simulink model "mcb_pmsm_hall_offset_f28069m"  (R2024b)
settings: Solver=FixedStepDiscrete  StartTime=0.0  StopTime=2  RelTol=1e-3  EnableMultiTasking=on
InitFcn:
  | mcb_pmsm_offset_data;
  | target = mcb_SetProcessorDetails('F28069M',PWM_frequency);
undefined symbols (not defined in the file): Down, GPTRIP1SEL, GPTRIP2SEL, motor, PWM_frequency, Ts, TZ1, TZ2, Up
libraries: simulink x8, idelinklib_common x6, svdschedulerlib x5, c280xlib x5, mcbcontrolslib x5, mcbpositiondecoderlib x4, c2802xlib x4, c2806xlib x2
(part 2 of 2)

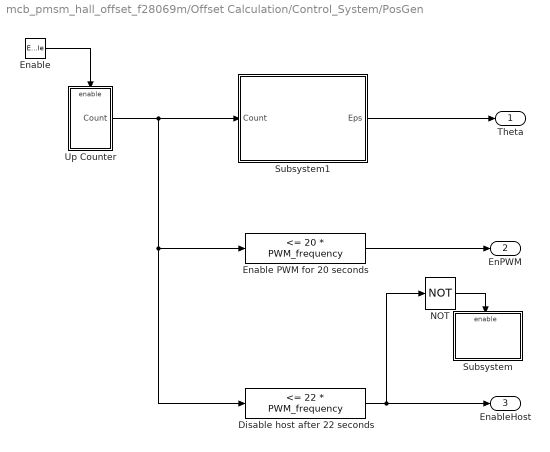
== system mcb_pmsm_hall_offset_f28069m/Offset Calculation/Control_System/PosGen ==
  Enable : EnablePort  StatesWhenEnabling=reset  ShowOutputPort=on
  Disable host after 22 seconds : simulink/Logic and Bit Operations/Compare To Constant  relop=<=  const=22 * PWM_frequency  OutDataTypeStr=boolean
  Enable PWM for 20 seconds : simulink/Logic and Bit Operations/Compare To Constant  relop=<=  const=20 * PWM_frequency  OutDataTypeStr=boolean
  NOT : Logic  Operator=NOT  IconShape=distinctive  AllPortsSameDT=off  OutDataTypeStr=boolean
  Subsystem : Subsystem
  Subsystem1 : Subsystem
  Up Counter : Subsystem
  Theta : Outport
  EnPWM : Outport  Port=2  OutputWhenDisabled=reset  InitialOutput=0  VectorParamsAs1DForOutWhenUnconnected=off
  EnableHost : Outport  Port=3  OutputWhenDisabled=reset  InitialOutput=0  VectorParamsAs1DForOutWhenUnconnected=off
  wires:
  Subsystem1/1(Eps) -> Theta/1
  Up Counter/1(Count) -> Disable host after 22 seconds/1, Enable PWM for 20 seconds/1, Subsystem1/1(Count)
  Enable/1 -> Up Counter/Enable
  NOT/1 -> Subsystem/Enable
  Enable PWM for 20 seconds/1 -> EnPWM/1
  Disable host after 22 seconds/1 -> NOT/1, EnableHost/1

== system mcb_pmsm_hall_offset_f28069m/Offset Calculation/Control_System/Subsystem1 ==
  Input : Inport
  Enable : EnablePort
  Offset : Outport
  wires:
  Input/1 -> Offset/1

== system mcb_pmsm_hall_offset_f28069m/Offset Calculation/Data Serial Output/Data ==
  Data : Inport
  Data_width : Inport  Port=2
  Action Port : ActionPort  ActionPortLabel=else
  Mux : Mux  Inputs=2
  Start : Constant  Value=hex2dec('0000')  OutDataTypeStr=uint16
  Data_out : Outport  VectorParamsAs1DForOutWhenUnconnected=off
  Iteration : Outport  Port=2  VectorParamsAs1DForOutWhenUnconnected=off
  wires:
  Start/1 -> Mux/2
  Mux/1 -> Data_out/1
  Data/1 -> Mux/1
  Data_width/1 -> Iteration/1

== system mcb_pmsm_hall_offset_f28069m/Offset Calculation/Data Serial Output/Data_Conditioning ==
  In1 : Inport
  Data Type Conversion1 : DataTypeConversion  OutDataTypeStr=fixdt(1,32,12)  RndMeth=Simplest  SaturateOnIntegerOverflow=off
  Data Type Conversion3 : DataTypeConversion  OutDataTypeStr=uint16  ConvertRealWorld=Stored Integer (SI)  SaturateOnIntegerOverflow=off  RndMeth=Floor
  Out1 : Outport
  wires:
  Data Type Conversion1/1 -> Data Type Conversion3/1
  In1/1 -> Data Type Conversion1/1
  Data Type Conversion3/1 -> Out1/1

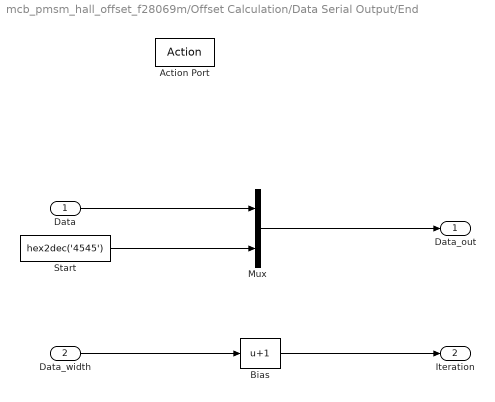
== system mcb_pmsm_hall_offset_f28069m/Offset Calculation/Data Serial Output/End ==
  Data : Inport
  Data_width : Inport  Port=2
  Action Port : ActionPort  ActionPortLabel=elseif(u1 == 599)
  Bias : Bias  Bias=1  SaturateOnIntegerOverflow=off
  Mux : Mux  Inputs=2
  Start : Constant  Value=hex2dec('4545')  OutDataTypeStr=uint16
  Data_out : Outport  VectorParamsAs1DForOutWhenUnconnected=off
  Iteration : Outport  Port=2  VectorParamsAs1DForOutWhenUnconnected=off
  wires:
  Mux/1 -> Data_out/1
  Data_width/1 -> Bias/1
  Start/1 -> Mux/2
  Bias/1 -> Iteration/1
  Data/1 -> Mux/1

== system mcb_pmsm_hall_offset_f28069m/Offset Calculation/Data Serial Output/Start ==
  Data : Inport
  Data_width : Inport  Port=2
  Action Port : ActionPort  ActionPortLabel=if(u1 == 0)
  Bias : Bias  Bias=1  SaturateOnIntegerOverflow=off
  End : Constant  Value=hex2dec('5353')  OutDataTypeStr=uint16
  Mux : Mux  Inputs=2
  Data_out : Outport  VectorParamsAs1DForOutWhenUnconnected=off
  Iteration : Outport  Port=2  VectorParamsAs1DForOutWhenUnconnected=off
  wires:
  End/1 -> Mux/1
  Mux/1 -> Data_out/1
  Data_width/1 -> Bias/1
  Bias/1 -> Iteration/1
  Data/1 -> Mux/2

== system mcb_pmsm_hall_offset_f28069m/Offset Calculation/Data Serial Output/While Iterator Subsystem ==
  Data : Inport
  Iteration : Inport  Port=2
  Add : Sum  Inputs=+-  OutDataTypeStr=Inherit: Same as first input
  Index Vector : MultiPortSwitch  Inputs=1  SaturateOnIntegerOverflow=off  InputSameDT=off
  SCI Transmit : c280xlib/SCI Transmit  sciModule=A  dataHead=''  dataTail=''  frameSize=1  blockingMode=on  outputStatus=off
  While Iterator : WhileIterator  MaxIters=-1  WhileBlockType=do-while  ShowIterationPort=on  OutputDataType=int16
  wires:
  Iteration/1 -> Add/1
  Add/1 -> While Iterator/1
  Index Vector/1 -> SCI Transmit/1
  Data/1 -> Index Vector/2
  While Iterator/1 -> Index Vector/1, Add/2

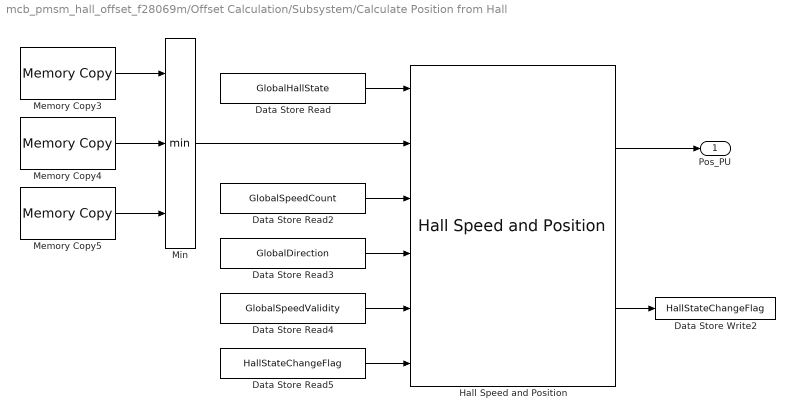
== system mcb_pmsm_hall_offset_f28069m/Offset Calculation/Subsystem/Calculate Position from Hall ==
  Data Store Read : DataStoreRead  DataStoreName=GlobalHallState  IndexOptions=Index vector (dialog)  Indices=1  OutputSizes=1
  Data Store Read2 : DataStoreRead  DataStoreName=GlobalSpeedCount  IndexOptions=Index vector (dialog)  Indices=1  OutputSizes=1
  Data Store Read3 : DataStoreRead  DataStoreName=GlobalDirection  IndexOptions=Index vector (dialog)  Indices=1  OutputSizes=1
  Data Store Read4 : DataStoreRead  DataStoreName=GlobalSpeedValidity  IndexOptions=Index vector (dialog)  Indices=1  OutputSizes=1
  Data Store Read5 : DataStoreRead  Priority=1  DataStoreName=HallStateChangeFlag  IndexOptions=Index vector (dialog)  Indices=1  OutputSizes=1
  Data Store Write2 : DataStoreWrite  Priority=2  DataStoreName=HallStateChangeFlag  IndexOptions=Index vector (dialog)  Indices=1  OutputSizes=1
  Hall Speed and Position : mcbpositiondecoderlib/Hall Speed and Position  blkExecutionType=Position  CounterSize=32 bits  ClkFreq=target.CPU_frequency  BlkSampleTime=Ts  PolePairs=motor.polePairs  MinSpeed=20  HallInterruptConfig=Every 180 Degrees  SpeedUnit=Per unit  PerUnitSpeed=6000  SpeedDataType=dataType  hallSequence=ABC  Sequence=[5,4,6,2,3,1]  EnableSecondOrder=1st Order  PositionUnit=Per unit  PositionDataType=dataType
  Memory Copy3 : idelinklib_common/Memory Copy  copyFrom=Specified source code symbol  copyFromAddressSource=Specify via dialog  copyFromAddress=hex2dec('00001000')  copyFromSrcCode=&ECap1Regs.TSCTR  dataTypeFrom=uint32  dataDimensionFrom=1  useOffsetFrom=off  offsetFromSrc=Specify via dialog  offsetFrom=0  strideFrom=1  copyTo=Output port  copyToAddressSource=Specify via dialog  copyToAddress=hex2dec('00002000')  copyToSrcCode=myVariableDst  dataTypeTo=uint32  useOffsetTo=off  offsetToSrc=Specify via dialog  offsetTo=0  strideTo=1  sampleTime=-1  useInitValue=off  initValueSrc=Specify constant value  initValue=1  initValueSrcCode=myInitValueVariable  useAsMask=off  maskOperator=bitwise AND  useTermValue=off  termValue=1  isRealtimeEnabled=off  emitCCBeforeWrite=off  CCBeforeWrite=/* Custom Code Before Write*/  emitCCAfterWrite=off  CCAfterWrite=/* Custom Code After Write*/
  Memory Copy4 : idelinklib_common/Memory Copy  copyFrom=Specified source code symbol  copyFromAddressSource=Specify via dialog  copyFromAddress=hex2dec('00001000')  copyFromSrcCode=&ECap2Regs.TSCTR  dataTypeFrom=uint32  dataDimensionFrom=1  useOffsetFrom=off  offsetFromSrc=Specify via dialog  offsetFrom=0  strideFrom=1  copyTo=Output port  copyToAddressSource=Specify via dialog  copyToAddress=hex2dec('00002000')  copyToSrcCode=myVariableDst  dataTypeTo=uint32  useOffsetTo=off  offsetToSrc=Specify via dialog  offsetTo=0  strideTo=1  sampleTime=-1  useInitValue=off  initValueSrc=Specify constant value  initValue=1  initValueSrcCode=myInitValueVariable  useAsMask=off  maskOperator=bitwise AND  useTermValue=off  termValue=1  isRealtimeEnabled=off  emitCCBeforeWrite=off  CCBeforeWrite=/* Custom Code Before Write*/  emitCCAfterWrite=off  CCAfterWrite=/* Custom Code After Write*/
  Memory Copy5 : idelinklib_common/Memory Copy  copyFrom=Specified source code symbol  copyFromAddressSource=Specify via dialog  copyFromAddress=hex2dec('00001000')  copyFromSrcCode=&ECap3Regs.TSCTR  dataTypeFrom=uint32  dataDimensionFrom=1  useOffsetFrom=off  offsetFromSrc=Specify via dialog  offsetFrom=0  strideFrom=1  copyTo=Output port  copyToAddressSource=Specify via dialog  copyToAddress=hex2dec('00002000')  copyToSrcCode=myVariableDst  dataTypeTo=uint32  useOffsetTo=off  offsetToSrc=Specify via dialog  offsetTo=0  strideTo=1  sampleTime=-1  useInitValue=off  initValueSrc=Specify constant value  initValue=1  initValueSrcCode=myInitValueVariable  useAsMask=off  maskOperator=bitwise AND  useTermValue=off  termValue=1  isRealtimeEnabled=off  emitCCBeforeWrite=off  CCBeforeWrite=/* Custom Code Before Write*/  emitCCAfterWrite=off  CCAfterWrite=/* Custom Code After Write*/
  Min : MinMax  Inputs=3
  Pos_PU : Outport  InitialOutput=0  VectorParamsAs1DForOutWhenUnconnected=off
  wires:
  Hall Speed and Position/2 -> Data Store Write2/1
  Data Store Read/1 -> Hall Speed and Position/1
  Data Store Read5/1 -> Hall Speed and Position/6
  Data Store Read4/1 -> Hall Speed and Position/5
  Memory Copy4/1 -> Min/2
  Min/1 -> Hall Speed and Position/2
  Memory Copy3/1 -> Min/1
  Data Store Read2/1 -> Hall Speed and Position/3
  Data Store Read3/1 -> Hall Speed and Position/4
  Memory Copy5/1 -> Min/3
  Hall Speed and Position/1 -> Pos_PU/1

== system mcb_pmsm_hall_offset_f28069m/Offset Calculation/Control_System/Find Offset/Subsystem ==
  Theta_hall : Inport
  Enable : EnablePort
  IIR Filter : mcbcontrolslib/IIR Filter  VariantControl=Low Pass Filter  VariantSelect=Low-pass  FilterConstantInputType=Specify via dialog  Filter_constant=0.5  advancedSettings=off  Ts=50e-6  cutOff_freq=3183.0989
  Offset : Outport
  wires:
  IIR Filter/1 -> Offset/1
  Theta_hall/1 -> IIR Filter/1

== system mcb_pmsm_hall_offset_f28069m/Offset Calculation/Control_System/PosGen/Subsystem ==
  Enable : EnablePort
  Constant : Constant  Value=0  OutDataTypeStr=Inherit: Inherit via back propagation
  Data Store Write : DataStoreWrite  DataStoreName=Enable  IndexOptions=Index vector (dialog)  Indices=1  OutputSizes=1
  wires:
  Constant/1 -> Data Store Write/1

== system mcb_pmsm_hall_offset_f28069m/Offset Calculation/Control_System/PosGen/Subsystem1 ==
  Count : Inport
  Count for 2 sec : Constant  Value=2.5 * PWM_frequency  OutDataTypeStr=uint32  SampleTime=-1
  If : If  NumInputs=2  IfExpression=u1 < u2
  If Action Subsystem : Subsystem  TreatAsAtomicUnit=on
  If Action Subsystem2 : Subsystem  TreatAsAtomicUnit=on
  Merge : Merge
  Position Generator : mcbcontrolslib/Position Generator  AngleOutput=Per-unit  ExternalReset=none  Offset=0
  Eps : Outport
  wires:
  If Action Subsystem/1(Out1) -> Merge/1
  If/1 -> If Action Subsystem/Action
  If Action Subsystem2/1(Out1) -> Merge/2
  Position Generator/1 -> Eps/1  "Eps"
  Count/1 -> If/1
  Merge/1 -> Position Generator/1
  If/2 -> If Action Subsystem2/Action
  Count for 2 sec/1 -> If/2

== system mcb_pmsm_hall_offset_f28069m/Offset Calculation/Control_System/PosGen/Up Counter ==
  Enable : EnablePort  StatesWhenEnabling=reset
  Add1 : Sum  SaturateOnIntegerOverflow=on
  Constant : Constant  OutDataTypeStr=uint32
  Delay : Delay  DelayLength=1
  Count : Outport  OutputWhenDisabled=reset  InitialOutput=0
  wires:
  Add1/1 -> Count/1, Delay/1
  Constant/1 -> Add1/1
  Delay/1 -> Add1/2

== system mcb_pmsm_hall_offset_f28069m/Offset Calculation/Control_System/PosGen/Subsystem1/If Action Subsystem ==
  Action Port : ActionPort  ActionPortLabel=if(u1 < u2)
  Constant : Constant  Value=0  OutDataTypeStr=dataType
  Out1 : Outport
  wires:
  Constant/1 -> Out1/1

== system mcb_pmsm_hall_offset_f28069m/Offset Calculation/Control_System/PosGen/Subsystem1/If Action Subsystem2 ==
  Action Port : ActionPort  ActionPortLabel=else
  Add1 : Sum
  Constant1 : Constant  Value=1e-3  OutDataTypeStr=dataType
  Delay : Delay  DelayLength=1
  Multiply : Gain  Gain=Ts  OutDataTypeStr=Inherit: Same as input
  Saturate to 'motor.calibSpeed' RPM : Saturate  UpperLimit=motor.polePairs * motor.calibSpeed / 60  LowerLimit=0
  Out1 : Outport
  wires:
  Delay/1 -> Add1/2
  Constant1/1 -> Add1/1
  Add1/1 -> Saturate to 'motor.calibSpeed' RPM/1
  Saturate to 'motor.calibSpeed' RPM/1 -> Delay/1, Multiply/1
  Multiply/1 -> Out1/1
